simulink model "PF_SeriesHybrid_SeriesParallelPartialHybrid_wDCDCReg"  (R2021b)
settings: Solver=FixedStepAuto  StartTime=0.0  StopTime=10  FixedStep=0.02  RelTol=1e-3
libraries: Lib_EMTAT x16, slpidlib x4
settings Model: Creator=sbianco1  LastModifiedBy=sbianco1
settings SolverCC: AlgebraicLoopSolver=TrustRegion
settings DebuggingCC: SFMachineParentedDataDiag=warning

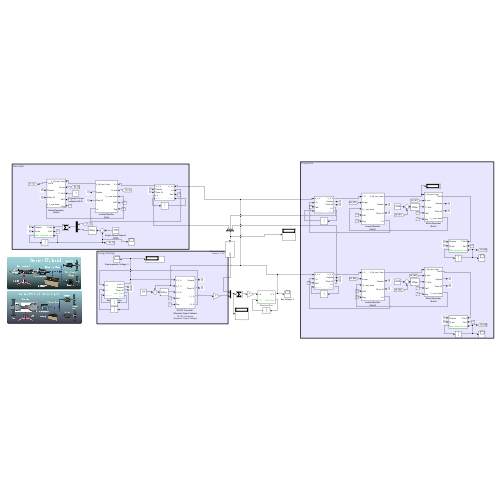
[thumbnail: Simulink's stored preview of the top-level diagram]
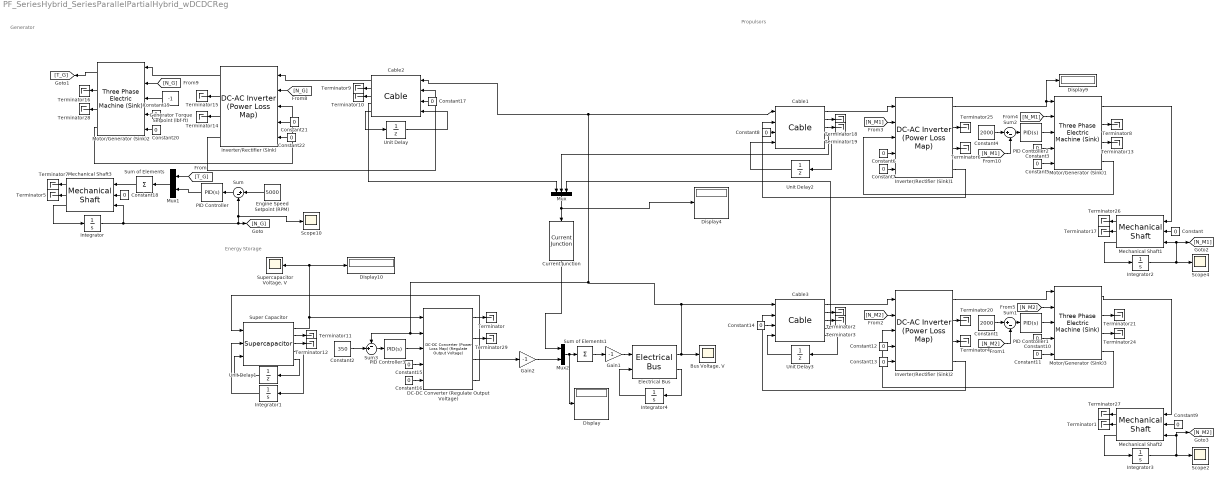
== system PF_SeriesHybrid_SeriesParallelPartialHybrid_wDCDCReg ==
  note: Propulsors
  note: Energy Storage
  note: Generator
  "Bus Voltage, V" : Scope
  Cable1 : Lib_EMTAT/Components/Power Flow/Cable  R=0.2
  Cable2 : Lib_EMTAT/Components/Power Flow/Cable  R=0.2
  Cable3 : Lib_EMTAT/Components/Power Flow/Cable  R=0.2
  Constant{,3,5..22} (20 alike) : Constant  Value=0
  Constant1 : Constant  Value=2000
  Constant2 : Constant  Value=350
  Constant4 : Constant  Value=2000
  Current Junction : Lib_EMTAT/Components/Power Flow/Current Junction  Nb=1
      settings: AttributesFormatString=|
      | Current Junction
      | Version: %<LibraryVersion>
  DC-DC Converter (Regulate Output Voltage) : Lib_EMTAT/Components/Power Flow/DC-DC Converter (Power Loss Map) (Regulate Output Voltage)  X_Vin_VoltageVec_M=[0 100 1000 5000]  Y_Iout_CurrentVec_M=[0 10 100 150]  T_C_PlossArray_M=100*ones(4,4)  FM=0  Plosslim=0
      settings: AttributesFormatString=|
      | DC-DC Converter
      | (Regulate Output Voltage)
  Display{,4,9..10} (4 alike) : Display
  Electrical Bus : Lib_EMTAT/Components/Power Flow/Electrical Bus  C=6e-3  Nb=1
      settings: AttributesFormatString=Electrical Bus
  Engine Speed Setpoint (RPM) : Constant  Value=5000
  Gain1 : Gain  Gain=-1
  Gain2 : Gain  Gain=-1
  Generator Torque Setpoint (lbf-ft) : Constant  Value=-1
  Integrator : Integrator  InitialCondition=5000
  Integrator1 : Integrator  InitialCondition=150
  Integrator2 : Integrator  InitialCondition=2000
  Integrator3 : Integrator  InitialCondition=2000
  Integrator4 : Integrator  InitialCondition=350
  Inverter/Rectifier (Sink) : Lib_EMTAT/Components/Power Flow/DC-AC Inverter (Power Loss Map)  X_C_VoltageInVec_M=[0 1000]  Y_C_RMSCurrentOutVec_M=[0 1000]  T_C_PowLossArray_M=100*ones(2)  K_e=0.0503  FM=0  Plosslim=0
  Inverter/Rectifier (Sink)1 : Lib_EMTAT/Components/Power Flow/DC-AC Inverter (Power Loss Map)  X_C_VoltageInVec_M=[0 1000]  Y_C_RMSCurrentOutVec_M=[0 1000]  T_C_PowLossArray_M=100*ones(2)  K_e=0.0503  FM=0  Plosslim=0
  Inverter/Rectifier (Sink)2 : Lib_EMTAT/Components/Power Flow/DC-AC Inverter (Power Loss Map)  X_C_VoltageInVec_M=[0 1000]  Y_C_RMSCurrentOutVec_M=[0 1000]  T_C_PowLossArray_M=100*ones(2)  K_e=0.0503  FM=0  Plosslim=0
  Mechanical Shaft1 : Lib_EMTAT/Components/Power Flow/Mechanical Shaft  J=0.01  B=0.001
  Mechanical Shaft2 : Lib_EMTAT/Components/Power Flow/Mechanical Shaft  J=0.01  B=0.001
  Mechanical Shaft3 : Lib_EMTAT/Components/Power Flow/Mechanical Shaft  J=0.01  B=0.001
  Motor/Generator (Sink)1 : Lib_EMTAT/Components/Power Flow/Three Phase Electric Machine (Sink)  X_C_SpeedVec_M=[0 100 1000 5000]  Y_C_TorqueVec_M=[0 10 100 150]  T_C_EffArray_M=0.99*ones(4,4)  FM=0
  Motor/Generator (Sink)2 : Lib_EMTAT/Components/Power Flow/Three Phase Electric Machine (Sink)  X_C_SpeedVec_M=[0 100 1000 5000]  Y_C_TorqueVec_M=[0 10 100 150]  T_C_EffArray_M=0.99*ones(4,4)  FM=0
  Motor/Generator (Sink)3 : Lib_EMTAT/Components/Power Flow/Three Phase Electric Machine (Sink)  X_C_SpeedVec_M=[0 100 1000 5000]  Y_C_TorqueVec_M=[0 10 100 150]  T_C_EffArray_M=0.99*ones(4,4)  FM=0
  Mux : Mux  Inputs=3
  Mux1 : Mux  Inputs=2
  Mux2 : Mux  Inputs=2
  PID Controller : slpidlib/PID Controller  Controller=PID  Form=Parallel  TimeDomain=Continuous-time  UseExternalTs=off  SampleTime=-1  IntegratorMethod=Forward Euler  FilterMethod=Forward Euler  ControllerParametersSource=internal  P=0.01  I=0.01  D=0  N=100  UseFilter=on  TunerSelectOption=Transfer Function Based (PID Tuner App)  InitialConditionSource=internal  InitialConditionForIntegrator=0  InitialConditionForFilter=0  DifferentiatorICPrevScaledInput=0  ExternalReset=none  TrackingMode=off  Kt=1  LimitOutput=off  SatLimitsSource=internal  UpperSaturationLimit=inf  LowerSaturationLimit=-inf  LinearizeAsGain=on  AntiWindupMode=none  Kb=1  POutMin=[]  POutMax=[]  IOutMin=[]  IOutMax=[]  DOutMin=[]  DOutMax=[]  NOutMin=[]  NOutMax=[]  SumOutMin=[]  SumOutMax=[]  SaturationOutMin=[]  SaturationOutMax=[]  PParamMin=[]  PParamMax=[]  IParamMin=[]  IParamMax=[]  DParamMin=[]  DParamMax=[]  NParamMin=[]  NParamMax=[]  KbParamMin=[]  KbParamMax=[]  KtParamMin=[]  KtParamMax=[]  KbOutMin=[]  KbOutMax=[]  KtOutMin=[]  KtOutMax=[]  IntegratorOutMin=[]  IntegratorOutMax=[]  FilterOutMin=[]  FilterOutMax=[]  SumI1OutMin=[]  SumI1OutMax=[]  SumI2OutMin=[]  SumI2OutMax=[]  SumI3OutMin=[]  SumI3OutMax=[]  SumI4OutMin=[]  SumI4OutMax=[]  SumDOutMin=[]  SumDOutMax=[]  DifferentiatorOutMin=[]  DifferentiatorOutMax=[]  FilterDiffOutCoefMin=[]  FilterDiffOutCoefMax=[]  ReciprocalOutMin=[]  ReciprocalOutMax=[]  SumDenOutMin=[]  SumDenOutMax=[]  SumNumOutMin=[]  SumNumOutMax=[]  DivideOutMin=[]  DivideOutMax=[]  UdiffTsProdOutMin=[]  UdiffTsProdOutMax=[]  NTsProdOutMin=[]  NTsProdOutMax=[]  UintegralTsProdOutMin=[]  UintegralTsProdOutMax=[]  UngainTsProdOutMin=[]  UngainTsProdOutMax=[]  IntegratorContinuousStateAttributes=''  IntegratorStateMustResolveToSignalObject=off  IntegratorRTWStateStorageClass=Auto  FilterContinuousStateAttributes=''  FilterStateMustResolveToSignalObject=off  FilterRTWStateStorageClass=Auto  ParallelPVariant=InternalParameters  IdealPVariant=Disabled  IVariant=InternalParameters  DVariant=InternalParameters  IntegratorVariant=Continuous  SatVariant=Disabled  AWVariant=Passthrough  PCopyVariant=Disabled  TRVariant=Disabled  FdbkBlocksVariant=Forward  IdealPFdbkVariant=Disabled  SatFdbkVariant=Disabled  DerivativeFilterVariant=ContFilter  NVariant=InternalParameters  NCopyVariant=Disabled  FilterICVariant=InternalICsFilter  IntegratorICVariant=InternalICs  ExternalResetVariant=Disabled  TRSumVariant=Passthrough  SumFdbkVariant=Disabled  SumVariant=Sum_PID  TsampFilterVariant=InternalTs  TsampNgainVariant=Passthrough  TsampIntegralVariant=Passthrough  ExternalSaturationOutDataTypeStr=Inherit: Same as second input
  PID Controller1 : slpidlib/PID Controller  Controller=PID  Form=Parallel  TimeDomain=Continuous-time  UseExternalTs=off  SampleTime=-1  IntegratorMethod=Forward Euler  FilterMethod=Forward Euler  ControllerParametersSource=internal  P=0.01  I=0.01  D=0  N=100  UseFilter=on  TunerSelectOption=Transfer Function Based (PID Tuner App)  InitialConditionSource=internal  InitialConditionForIntegrator=0  InitialConditionForFilter=0  DifferentiatorICPrevScaledInput=0  ExternalReset=none  TrackingMode=off  Kt=1  LimitOutput=off  SatLimitsSource=internal  UpperSaturationLimit=inf  LowerSaturationLimit=-inf  LinearizeAsGain=on  AntiWindupMode=none  Kb=1  POutMin=[]  POutMax=[]  IOutMin=[]  IOutMax=[]  DOutMin=[]  DOutMax=[]  NOutMin=[]  NOutMax=[]  SumOutMin=[]  SumOutMax=[]  SaturationOutMin=[]  SaturationOutMax=[]  PParamMin=[]  PParamMax=[]  IParamMin=[]  IParamMax=[]  DParamMin=[]  DParamMax=[]  NParamMin=[]  NParamMax=[]  KbParamMin=[]  KbParamMax=[]  KtParamMin=[]  KtParamMax=[]  KbOutMin=[]  KbOutMax=[]  KtOutMin=[]  KtOutMax=[]  IntegratorOutMin=[]  IntegratorOutMax=[]  FilterOutMin=[]  FilterOutMax=[]  SumI1OutMin=[]  SumI1OutMax=[]  SumI2OutMin=[]  SumI2OutMax=[]  SumI3OutMin=[]  SumI3OutMax=[]  SumI4OutMin=[]  SumI4OutMax=[]  SumDOutMin=[]  SumDOutMax=[]  DifferentiatorOutMin=[]  DifferentiatorOutMax=[]  FilterDiffOutCoefMin=[]  FilterDiffOutCoefMax=[]  ReciprocalOutMin=[]  ReciprocalOutMax=[]  SumDenOutMin=[]  SumDenOutMax=[]  SumNumOutMin=[]  SumNumOutMax=[]  DivideOutMin=[]  DivideOutMax=[]  UdiffTsProdOutMin=[]  UdiffTsProdOutMax=[]  NTsProdOutMin=[]  NTsProdOutMax=[]  UintegralTsProdOutMin=[]  UintegralTsProdOutMax=[]  UngainTsProdOutMin=[]  UngainTsProdOutMax=[]  IntegratorContinuousStateAttributes=''  IntegratorStateMustResolveToSignalObject=off  IntegratorRTWStateStorageClass=Auto  FilterContinuousStateAttributes=''  FilterStateMustResolveToSignalObject=off  FilterRTWStateStorageClass=Auto  ParallelPVariant=InternalParameters  IdealPVariant=Disabled  IVariant=InternalParameters  DVariant=InternalParameters  IntegratorVariant=Continuous  SatVariant=Disabled  AWVariant=Passthrough  PCopyVariant=Disabled  TRVariant=Disabled  FdbkBlocksVariant=Forward  IdealPFdbkVariant=Disabled  SatFdbkVariant=Disabled  DerivativeFilterVariant=ContFilter  NVariant=InternalParameters  NCopyVariant=Disabled  FilterICVariant=InternalICsFilter  IntegratorICVariant=InternalICs  ExternalResetVariant=Disabled  TRSumVariant=Passthrough  SumFdbkVariant=Disabled  SumVariant=Sum_PID  TsampFilterVariant=InternalTs  TsampNgainVariant=Passthrough  TsampIntegralVariant=Passthrough  ExternalSaturationOutDataTypeStr=Inherit: Same as second input
  PID Controller2 : slpidlib/PID Controller  Controller=PID  Form=Parallel  TimeDomain=Continuous-time  UseExternalTs=off  SampleTime=-1  IntegratorMethod=Forward Euler  FilterMethod=Forward Euler  ControllerParametersSource=internal  P=0.01  I=0.01  D=0  N=100  UseFilter=on  TunerSelectOption=Transfer Function Based (PID Tuner App)  InitialConditionSource=internal  InitialConditionForIntegrator=0  InitialConditionForFilter=0  DifferentiatorICPrevScaledInput=0  ExternalReset=none  TrackingMode=off  Kt=1  LimitOutput=off  SatLimitsSource=internal  UpperSaturationLimit=inf  LowerSaturationLimit=-inf  LinearizeAsGain=on  AntiWindupMode=none  Kb=1  POutMin=[]  POutMax=[]  IOutMin=[]  IOutMax=[]  DOutMin=[]  DOutMax=[]  NOutMin=[]  NOutMax=[]  SumOutMin=[]  SumOutMax=[]  SaturationOutMin=[]  SaturationOutMax=[]  PParamMin=[]  PParamMax=[]  IParamMin=[]  IParamMax=[]  DParamMin=[]  DParamMax=[]  NParamMin=[]  NParamMax=[]  KbParamMin=[]  KbParamMax=[]  KtParamMin=[]  KtParamMax=[]  KbOutMin=[]  KbOutMax=[]  KtOutMin=[]  KtOutMax=[]  IntegratorOutMin=[]  IntegratorOutMax=[]  FilterOutMin=[]  FilterOutMax=[]  SumI1OutMin=[]  SumI1OutMax=[]  SumI2OutMin=[]  SumI2OutMax=[]  SumI3OutMin=[]  SumI3OutMax=[]  SumI4OutMin=[]  SumI4OutMax=[]  SumDOutMin=[]  SumDOutMax=[]  DifferentiatorOutMin=[]  DifferentiatorOutMax=[]  FilterDiffOutCoefMin=[]  FilterDiffOutCoefMax=[]  ReciprocalOutMin=[]  ReciprocalOutMax=[]  SumDenOutMin=[]  SumDenOutMax=[]  SumNumOutMin=[]  SumNumOutMax=[]  DivideOutMin=[]  DivideOutMax=[]  UdiffTsProdOutMin=[]  UdiffTsProdOutMax=[]  NTsProdOutMin=[]  NTsProdOutMax=[]  UintegralTsProdOutMin=[]  UintegralTsProdOutMax=[]  UngainTsProdOutMin=[]  UngainTsProdOutMax=[]  IntegratorContinuousStateAttributes=''  IntegratorStateMustResolveToSignalObject=off  IntegratorRTWStateStorageClass=Auto  FilterContinuousStateAttributes=''  FilterStateMustResolveToSignalObject=off  FilterRTWStateStorageClass=Auto  ParallelPVariant=InternalParameters  IdealPVariant=Disabled  IVariant=InternalParameters  DVariant=InternalParameters  IntegratorVariant=Continuous  SatVariant=Disabled  AWVariant=Passthrough  PCopyVariant=Disabled  TRVariant=Disabled  FdbkBlocksVariant=Forward  IdealPFdbkVariant=Disabled  SatFdbkVariant=Disabled  DerivativeFilterVariant=ContFilter  NVariant=InternalParameters  NCopyVariant=Disabled  FilterICVariant=InternalICsFilter  IntegratorICVariant=InternalICs  ExternalResetVariant=Disabled  TRSumVariant=Passthrough  SumFdbkVariant=Disabled  SumVariant=Sum_PID  TsampFilterVariant=InternalTs  TsampNgainVariant=Passthrough  TsampIntegralVariant=Passthrough  ExternalSaturationOutDataTypeStr=Inherit: Same as second input
  PID Controller3 : slpidlib/PID Controller  Controller=PID  Form=Parallel  TimeDomain=Continuous-time  UseExternalTs=off  SampleTime=-1  IntegratorMethod=Forward Euler  FilterMethod=Forward Euler  ControllerParametersSource=internal  P=1  I=1  D=0  N=100  UseFilter=on  TunerSelectOption=Transfer Function Based (PID Tuner App)  InitialConditionSource=internal  InitialConditionForIntegrator=0  InitialConditionForFilter=0  DifferentiatorICPrevScaledInput=0  ExternalReset=none  TrackingMode=off  Kt=1  LimitOutput=off  SatLimitsSource=internal  UpperSaturationLimit=inf  LowerSaturationLimit=-inf  LinearizeAsGain=on  AntiWindupMode=none  Kb=1  POutMin=[]  POutMax=[]  IOutMin=[]  IOutMax=[]  DOutMin=[]  DOutMax=[]  NOutMin=[]  NOutMax=[]  SumOutMin=[]  SumOutMax=[]  SaturationOutMin=[]  SaturationOutMax=[]  PParamMin=[]  PParamMax=[]  IParamMin=[]  IParamMax=[]  DParamMin=[]  DParamMax=[]  NParamMin=[]  NParamMax=[]  KbParamMin=[]  KbParamMax=[]  KtParamMin=[]  KtParamMax=[]  KbOutMin=[]  KbOutMax=[]  KtOutMin=[]  KtOutMax=[]  IntegratorOutMin=[]  IntegratorOutMax=[]  FilterOutMin=[]  FilterOutMax=[]  SumI1OutMin=[]  SumI1OutMax=[]  SumI2OutMin=[]  SumI2OutMax=[]  SumI3OutMin=[]  SumI3OutMax=[]  SumI4OutMin=[]  SumI4OutMax=[]  SumDOutMin=[]  SumDOutMax=[]  DifferentiatorOutMin=[]  DifferentiatorOutMax=[]  FilterDiffOutCoefMin=[]  FilterDiffOutCoefMax=[]  ReciprocalOutMin=[]  ReciprocalOutMax=[]  SumDenOutMin=[]  SumDenOutMax=[]  SumNumOutMin=[]  SumNumOutMax=[]  DivideOutMin=[]  DivideOutMax=[]  UdiffTsProdOutMin=[]  UdiffTsProdOutMax=[]  NTsProdOutMin=[]  NTsProdOutMax=[]  UintegralTsProdOutMin=[]  UintegralTsProdOutMax=[]  UngainTsProdOutMin=[]  UngainTsProdOutMax=[]  IntegratorContinuousStateAttributes=''  IntegratorStateMustResolveToSignalObject=off  IntegratorRTWStateStorageClass=Auto  FilterContinuousStateAttributes=''  FilterStateMustResolveToSignalObject=off  FilterRTWStateStorageClass=Auto  ParallelPVariant=InternalParameters  IdealPVariant=Disabled  IVariant=InternalParameters  DVariant=InternalParameters  IntegratorVariant=Continuous  SatVariant=Disabled  AWVariant=Passthrough  PCopyVariant=Disabled  TRVariant=Disabled  FdbkBlocksVariant=Forward  IdealPFdbkVariant=Disabled  SatFdbkVariant=Disabled  DerivativeFilterVariant=ContFilter  NVariant=InternalParameters  NCopyVariant=Disabled  FilterICVariant=InternalICsFilter  IntegratorICVariant=InternalICs  ExternalResetVariant=Disabled  TRSumVariant=Passthrough  SumFdbkVariant=Disabled  SumVariant=Sum_PID  TsampFilterVariant=InternalTs  TsampNgainVariant=Passthrough  TsampIntegralVariant=Passthrough  ExternalSaturationOutDataTypeStr=Inherit: Same as second input
  Scope10 : Scope
  Scope2 : Scope
  Scope4 : Scope
  Sum : Sum  Inputs=|+-
  Sum of Elements : Sum  Inputs=+
  Sum of Elements1 : Sum  Inputs=+
  Sum1 : Sum  Inputs=|+-
  Sum2 : Sum  Inputs=|+-
  Sum3 : Sum  Inputs=-+|
  Super Capacitor : Lib_EMTAT/Components/Power Flow/Supercapacitor  C=130  ESR=0.02  TSE=200  BlkNm=double(gcb)
  "Supercapacitor Voltage, V" : Scope
  Terminator{,1..21,24..29} (28 alike) : Terminator
  Unit Delay{,1..3} (4 alike) : UnitDelay  SampleTime=-1  HasFrameUpgradeWarning=on
  wires:
  Constant2/1 -> Sum3/2
  Super Capacitor/1 -> DC-DC Converter (Regulate Output Voltage)/1, Display10/1, "Supercapacitor Voltage, V"/1
  Current Junction/1 -> Mux2/1
  DC-DC Converter (Regulate Output Voltage)/4 -> Super Capacitor/1
  Inverter/Rectifier (Sink)/2 -> Terminator15/1
  Inverter/Rectifier (Sink)/1 -> Motor/Generator (Sink)2/1
  Inverter/Rectifier (Sink)/4 -> Cable2/2
  [N_G] -> Motor/Generator (Sink)2/2
  Motor/Generator (Sink)2/4 -> Inverter/Rectifier (Sink)/3
  Cable2/1 -> Inverter/Rectifier (Sink)/1
  Inverter/Rectifier (Sink)/3 -> Terminator14/1
  [N_G] -> Inverter/Rectifier (Sink)/2
  Motor/Generator (Sink)2/2 -> Terminator16/1
  Generator Torque Setpoint (lbf-ft)/1 -> Motor/Generator (Sink)2/3
  Mux/1 -> Current Junction/1, Display4/1
  PID Controller2/1 -> Motor/Generator (Sink)1/3
  Sum2/1 -> PID Controller2/1
  Motor/Generator (Sink)1/2 -> Terminator8/1
  Cable1/4 -> Mux/2
  [N_M1] -> Sum2/2
  Constant4/1 -> Sum2/1
  [N_M1] -> Motor/Generator (Sink)1/2
  Cable1/1 -> Inverter/Rectifier (Sink)1/1
  Motor/Generator (Sink)1/1 -> Mechanical Shaft1/1
  Inverter/Rectifier (Sink)1/1 -> Motor/Generator (Sink)1/1, Display9/1
  Inverter/Rectifier (Sink)1/4 -> Cable1/2
  Mechanical Shaft1/2 -> Terminator17/1
  [N_M1] -> Inverter/Rectifier (Sink)1/2
  Inverter/Rectifier (Sink)1/3 -> Terminator6/1
  Cable2/4 -> Mux/1
  Cable2/2 -> Terminator9/1
  Cable2/3 -> Terminator10/1
  Super Capacitor/2 -> Terminator11/1
  Super Capacitor/3 -> Terminator12/1
  Cable1/2 -> Terminator18/1
  Cable1/3 -> Terminator19/1
  Inverter/Rectifier (Sink)2/3 -> Terminator4/1
  Cable3/3 -> Terminator3/1
  [N_M2] -> Sum1/2
  Sum1/1 -> PID Controller1/1
  [N_M2] -> Motor/Generator (Sink)3/2
  Motor/Generator (Sink)3/2 -> Terminator21/1
  Inverter/Rectifier (Sink)2/4 -> Cable3/2
  Inverter/Rectifier (Sink)2/2 -> Terminator20/1
  Cable3/2 -> Terminator2/1
  Cable3/1 -> Inverter/Rectifier (Sink)2/1
  Motor/Generator (Sink)3/1 -> Mechanical Shaft2/1
  [N_M2] -> Inverter/Rectifier (Sink)2/2
  Mechanical Shaft2/2 -> Terminator1/1
  Cable3/4 -> Mux/3
  Constant1/1 -> Sum1/1
  Inverter/Rectifier (Sink)2/1 -> Motor/Generator (Sink)3/1
  Electrical Bus/1 -> "Bus Voltage, V"/1, Sum3/1, DC-DC Converter (Regulate Output Voltage)/2, Cable2/1, Cable1/1, Cable3/1
  Mechanical Shaft3/2 -> Terminator5/1
  Motor/Generator (Sink)2/1 -> [T_G]
  Mux1/1 -> Sum of Elements/1
  [T_G] -> Mux1/1
  Integrator/1 -> Mechanical Shaft3/3, Sum/2, Scope10/1, [N_G]
  PID Controller/1 -> Mux1/2
  Sum/1 -> PID Controller/1
  Engine Speed Setpoint (RPM)/1 -> Sum/1
  Cable2/5 -> Unit Delay/1
  Super Capacitor/5 -> Unit Delay1/1
  Unit Delay1/1 -> Super Capacitor/3
  Integrator1/1 -> Super Capacitor/2
  Super Capacitor/4 -> Integrator1/1
  Cable1/5 -> Unit Delay2/1
  Unit Delay2/1 -> Cable1/4
  Cable3/5 -> Unit Delay3/1
  Unit Delay3/1 -> Cable3/4
  Integrator2/1 -> Scope4/1, [N_M1], Mechanical Shaft1/3
  Integrator3/1 -> Scope2/1, [N_M2], Mechanical Shaft2/3
  Inverter/Rectifier (Sink)1/2 -> Terminator25/1
  Mechanical Shaft1/1 -> Terminator26/1
  Mechanical Shaft1/3 -> Integrator2/1
  Constant/1 -> Mechanical Shaft1/2
  Constant3/1 -> Motor/Generator (Sink)1/4
  Constant5/1 -> Motor/Generator (Sink)1/5
  Motor/Generator (Sink)1/3 -> Terminator13/1
  Motor/Generator (Sink)1/4 -> Inverter/Rectifier (Sink)1/3
  Constant6/1 -> Inverter/Rectifier (Sink)1/4
  Constant7/1 -> Inverter/Rectifier (Sink)1/5
  Constant8/1 -> Cable1/3
  Constant9/1 -> Mechanical Shaft2/2
  Mechanical Shaft2/1 -> Terminator27/1
  Mechanical Shaft2/3 -> Integrator3/1
  Motor/Generator (Sink)3/3 -> Terminator24/1
  Motor/Generator (Sink)3/4 -> Inverter/Rectifier (Sink)2/3
  PID Controller1/1 -> Motor/Generator (Sink)3/3
  Constant10/1 -> Motor/Generator (Sink)3/4
  Constant11/1 -> Motor/Generator (Sink)3/5
  Constant12/1 -> Inverter/Rectifier (Sink)2/4
  Constant13/1 -> Inverter/Rectifier (Sink)2/5
  Constant14/1 -> Cable3/3
  Constant15/1 -> DC-DC Converter (Regulate Output Voltage)/4
  Constant16/1 -> DC-DC Converter (Regulate Output Voltage)/5
  Unit Delay/1 -> Cable2/4
  Constant17/1 -> Cable2/3
  Mechanical Shaft3/1 -> Terminator7/1
  Mechanical Shaft3/3 -> Integrator/1
  Constant18/1 -> Mechanical Shaft3/2
  Motor/Generator (Sink)2/3 -> Terminator28/1
  Constant19/1 -> Motor/Generator (Sink)2/4
  Constant20/1 -> Motor/Generator (Sink)2/5
  Constant21/1 -> Inverter/Rectifier (Sink)/4
  Constant22/1 -> Inverter/Rectifier (Sink)/5
  Sum of Elements/1 -> Mechanical Shaft3/1
  Mux2/1 -> Display/1, Sum of Elements1/1
  DC-DC Converter (Regulate Output Voltage)/3 -> Gain2/1
  DC-DC Converter (Regulate Output Voltage)/1 -> Terminator/1
  DC-DC Converter (Regulate Output Voltage)/2 -> Terminator29/1
  PID Controller3/1 -> DC-DC Converter (Regulate Output Voltage)/3
  Electrical Bus/2 -> Integrator4/1
  Integrator4/1 -> Electrical Bus/2
  Sum3/1 -> PID Controller3/1
  Sum of Elements1/1 -> Gain1/1
  Gain1/1 -> Electrical Bus/1
  Gain2/1 -> Mux2/2
